simulink model "modelSVPWM"  (R2024a)
settings: Solver=ode23tb  StartTime=0.0  StopTime=0.1  MaxStep=sover_max_step  RelTol=1e-5
values from neighbouring files (symbols this model uses):
  f_fundamental = 265    [initBCPWM.m]    (also in initSVPWM.m = 100)
  f_pwm = 20000    [initBCPWM.m]    (also in initSVPWM.m)
  Ke = sqrt(2) * 3.35e-3 * 60 / 2 / pi / p    [initBCPWM.m]    (also in initSVPWM.m)
  load_angle = pi/6    (= 0.523598775598)    [initBCPWM.m]    (also in initSVPWM.m = load_angle_offset - voltage_angle)
  Ls = 3/2 * 1.2e-3    (= 0.0018)    [initBCPWM.m]    (also in initSVPWM.m)
  Rs = 3/2 * 0.8    (= 1.2)    [initBCPWM.m]    (also in initSVPWM.m)
  sover_max_step = 1e-6    (= 1e-06)    [initBCPWM.m]    (also in initSVPWM.m)
  V_uvw = Vsetpoint    (= 5)    [initSVPWM.m]
  Vdc = 24    [initBCPWM.m]    (also in initSVPWM.m)
libraries: simulink x14, spsSeriesRLCBranchLib x6, spsVoltageMeasurementLib x6, spsMosfetLib x6, spsNeutralLib x5, spsControlledVoltageSourceLib x3, spsCurrentMeasurementLib x3, spsGroundLib x2, spsDCVoltageSourceLib x1, spspowerguiLib x1
settings Model: Creator=mandr  LastModifiedBy=danielmcguiness
settings SolverCC: ZeroCrossControl=EnableAll  AlgebraicLoopSolver=TrustRegion  SolverResetMethod=Robust
settings DebuggingCC: UnconnectedInputMsg=warning  UnconnectedOutputMsg=warning  UnconnectedLineMsg=warning
settings ModelReferenceCC: EnableRefExpFcnMdlSchedulingChecks=on
settings RTWCC: GPUComputeCapability=3.5

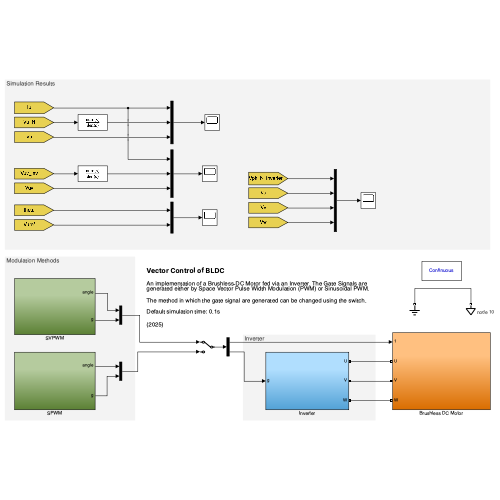
[thumbnail: Simulink's stored preview of the top-level diagram]
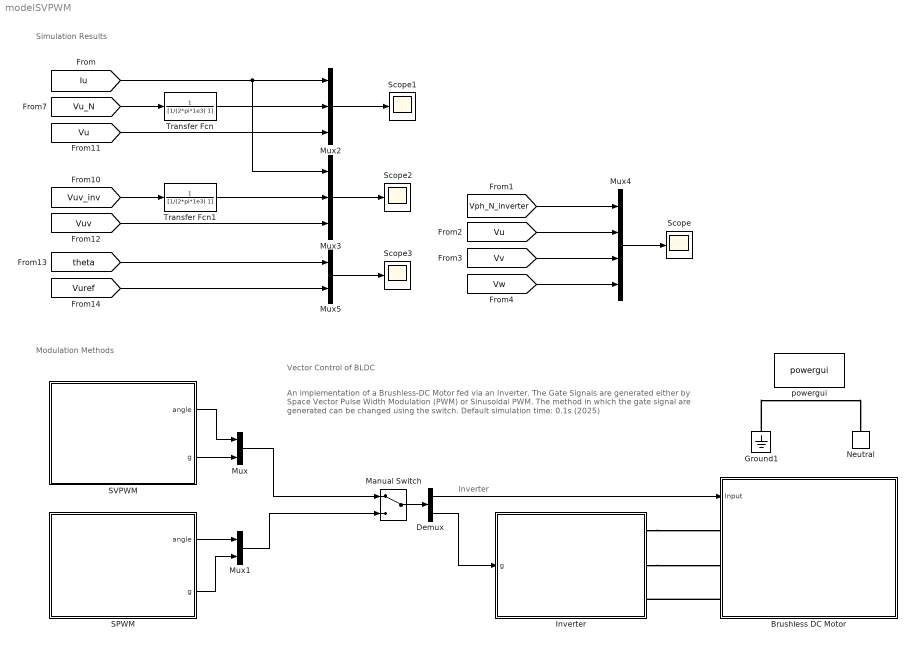
== system modelSVPWM ==
  note: Modulation Methods
  note: Simulation Results
  note: An implementation of a Brushless-DC Motor fed via an Inverter. The Gate Signals are generated either by Space Vector Pulse Width Modulation (PWM) or Sinusoidal PWM.
      |
      | The method in which the gate signal are generated can be changed using the switch.
      |
      | Default simulation time: 0.1s
      |
      | (2025)
  note: Vector Control of BLDC
  note: Inverter
  Brushless DC Motor : Subsystem
  Demux : Demux  Outputs=2
  Ground1 : spsGroundLib/Ground  LConnTagsString=a
  Inverter : Subsystem
  Manual Switch : ManualSwitch
  Mux : Mux  Inputs=2
  Mux1 : Mux  Inputs=2
  Mux2 : Mux  Inputs=3
  Mux3 : Mux  Inputs=3
  Mux4 : Mux
  Mux5 : Mux  Inputs=2
  Neutral : spsNeutralLib/Neutral  LConnTagsString=a  NodeNumber=10
      settings: AttributesFormatString=node %<NodeNumber>  LibrarySourceBlock=sps_lib/Utilities/Neutral
  SPWM : Subsystem
  SVPWM : Subsystem
  Scope{,1..3} (4 alike) : Scope
  Transfer Fcn : TransferFcn  Denominator=[1/(2*pi*1e3) 1]
  Transfer Fcn1 : TransferFcn  Denominator=[1/(2*pi*1e3) 1]
  powergui : spspowerguiLib/powergui  Priority=1  SimulationMode=Continuous  SampleTime=50e-6  frequency=60  Iterations=50  frequencyindice=0  Pbase=100e6  ErrMax=1e-4  UnitsV=kV  UnitsW=MW  buscounter=0  FunctionMessages=off  echomessages=off  EnableUseOfTLC=off  CurrentSourceSwitches=off  DisableSnubberDevices=off  DisableRonSwitches=off  DisableVfSwitches=off  DisplayEquations=off  AutomaticDiscreteSolvers=off  SolverType=Tustin/Backward Euler (TBE)  Interpol=off  ExternalGateDelay=off  methode=off  Ts=100  x0status=blocks  SPID=on  SwTol=0  HookPort=off  NonlinearTolerance=1e-4  nMaxIteration=100  ContinueOnMaxIteration=off  RestoreLinks=warning  ResistiveCurrentMeasurement=off  Frange=[0:2:500]  Ylog=off  Xlog=on  ShowGrid=off  save=off  variable=ZData  structure=0  ZoomFFT=off  StartTime=0.0  cycles=1  DisplayStyle=1  fundamental=60  FreqAxis=off  MaxFrequency=1000  frequencyindicesteady=1  RmsSteady=1  display=off
  wires:
  Mux/1 -> Manual Switch/1
  SVPWM/1(angle) -> Mux/1
  SVPWM/2(g) -> Mux/2
  Manual Switch/1 -> Demux/1
  Demux/2 -> Inverter/1(g)
  Demux/1 -> Brushless DC Motor/1(Input)
  SPWM/1(angle) -> Mux1/1
  SPWM/2(g) -> Mux1/2
  Mux1/1 -> Manual Switch/2
  [theta] -> Mux5/1
  Transfer Fcn/1 -> Mux2/2
  Mux2/1 -> Scope1/1
  [Vu_N] -> Transfer Fcn/1
  [Vuv] -> Mux3/3
  Transfer Fcn1/1 -> Mux3/2
  [Vuref] -> Mux5/2
  Mux3/1 -> Scope2/1
  [Vuv_inv] -> Transfer Fcn1/1
  [Vu] -> Mux2/3
  [Iu] -> Mux2/1, Mux3/1
  Mux4/1 -> Scope/1
  [Vw] -> Mux4/4
  [Vph_N_inverter] -> Mux4/1
  [Vv] -> Mux4/3
  [Vu] -> Mux4/2
  Mux5/1 -> Scope3/1
  connections:
  Inverter/RConn2 -- Brushless DC Motor/LConn2
  Brushless DC Motor/LConn3 -- Inverter/RConn3
  Inverter/RConn1 -- Brushless DC Motor/LConn1
  Ground1/LConn1 -- Neutral/LConn1

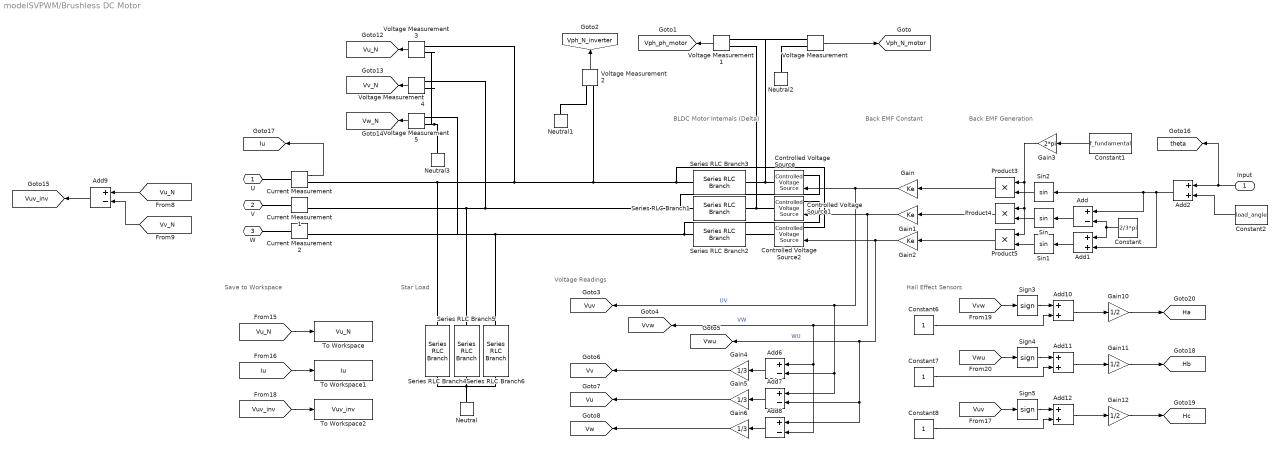
== system modelSVPWM/Brushless DC Motor ==
  note: Save to Workspace
  note: Star Load
  note: Back EMF Generation
  note: Back EMF Constant
  note: BLDC Motor Internals (Delta)
  note: Hall Effect Sensors
  note: Voltage Readings
  Input : Inport
  Add{,6..9} (5 alike) : Sum  Inputs=+-
  Add{1..2,10..12} (5 alike) : Sum
  Constant : Constant  Value=2/3*pi
  Constant1 : Constant  Value=f_fundamental
  Constant2 : Constant  Value=load_angle
  Constant6 : Constant
  Constant7 : Constant
  Constant8 : Constant
  Controlled Voltage Source : spsControlledVoltageSourceLib/Controlled Voltage Source  Initialize=on  Source_Type=AC  Amplitude=0  Phase=0  Frequency=0  Measurements=None
  Controlled Voltage Source1 : spsControlledVoltageSourceLib/Controlled Voltage Source  Initialize=on  Source_Type=AC  Amplitude=0  Phase=0  Frequency=0  Measurements=None
  Controlled Voltage Source2 : spsControlledVoltageSourceLib/Controlled Voltage Source  Initialize=on  Source_Type=AC  Amplitude=0  Phase=0  Frequency=0  Measurements=None
  Current Measurement : spsCurrentMeasurementLib/Current Measurement  PhasorSimulation=off  OutputType=Complex  PSBequivalent=0
  Current Measurement1 : spsCurrentMeasurementLib/Current Measurement  PhasorSimulation=off  OutputType=Complex  PSBequivalent=0
  Current Measurement2 : spsCurrentMeasurementLib/Current Measurement  PhasorSimulation=off  OutputType=Complex  PSBequivalent=0
  Gain : Gain  Gain=Ke
  Gain1 : Gain  Gain=Ke
  Gain10 : Gain  Gain=1/2
  Gain11 : Gain  Gain=1/2
  Gain12 : Gain  Gain=1/2
  Gain2 : Gain  Gain=Ke
  Gain3 : Gain  Gain=2*pi
  Gain4 : Gain  Gain=1/3
  Gain5 : Gain  Gain=1/3
  Gain6 : Gain  Gain=1/3
  Neutral{,1..3} (4 alike) : spsNeutralLib/Neutral  LConnTagsString=a  NodeNumber=10
      settings: AttributesFormatString=node %<NodeNumber>  LibrarySourceBlock=sps_lib/Utilities/Neutral
  Product3 : Product
  Product4 : Product
  Product5 : Product
  Series RLC Branch1 : spsSeriesRLCBranchLib/Series RLC Branch  LConnTagsString=__new0  RConnTagsString=__new0  BranchType=RL  Resistance=Rs  Inductance=Ls  SetiL0=off  InitialCurrent=0  Capacitance=1e-6  Setx0=off  InitialVoltage=0  Measurements=None
  Series RLC Branch2 : spsSeriesRLCBranchLib/Series RLC Branch  LConnTagsString=__new0  RConnTagsString=__new0  BranchType=RL  Resistance=Rs  Inductance=Ls  SetiL0=off  InitialCurrent=0  Capacitance=1e-6  Setx0=off  InitialVoltage=0  Measurements=None
  Series RLC Branch3 : spsSeriesRLCBranchLib/Series RLC Branch  LConnTagsString=__new0  RConnTagsString=__new0  BranchType=RL  Resistance=Rs  Inductance=Ls  SetiL0=off  InitialCurrent=0  Capacitance=1e-6  Setx0=off  InitialVoltage=0  Measurements=None
  Series RLC Branch4 : spsSeriesRLCBranchLib/Series RLC Branch  LConnTagsString=__new0  RConnTagsString=__new0  BranchType=R  Resistance=1e3  Inductance=Ls  SetiL0=off  InitialCurrent=0  Capacitance=1e-6  Setx0=off  InitialVoltage=0  Measurements=None
  Series RLC Branch5 : spsSeriesRLCBranchLib/Series RLC Branch  LConnTagsString=__new0  RConnTagsString=__new0  BranchType=R  Resistance=1e3  Inductance=Ls  SetiL0=off  InitialCurrent=0  Capacitance=1e-6  Setx0=off  InitialVoltage=0  Measurements=None
  Series RLC Branch6 : spsSeriesRLCBranchLib/Series RLC Branch  LConnTagsString=__new0  RConnTagsString=__new0  BranchType=R  Resistance=1e3  Inductance=Ls  SetiL0=off  InitialCurrent=0  Capacitance=1e-6  Setx0=off  InitialVoltage=0  Measurements=None
  Sign3 : Signum
  Sign4 : Signum
  Sign5 : Signum
  Sin : Trigonometry
  Sin1 : Trigonometry
  Sin2 : Trigonometry
  To Workspace : ToWorkspace  VariableName=Vu_N  SaveFormat=Timeseries  SampleTime=sover_max_step
  To Workspace1 : ToWorkspace  VariableName=Iu  SaveFormat=Timeseries  SampleTime=sover_max_step
  To Workspace2 : ToWorkspace  VariableName=Vuv_inv  SaveFormat=Timeseries  SampleTime=sover_max_step
  Voltage Measurement{,1..5} (6 alike) : spsVoltageMeasurementLib/Voltage Measurement  PhasorSimulation=off  OutputType=Complex  PSBequivalent=0
  U : PMIOPort  Side=Left
  V : PMIOPort  Port=2  Side=Left
  W : PMIOPort  Port=3  Side=Left
  tag scope: Ha=global, Hb=global, Hc=global, Iu=global, Vph_N_inverter=global, Vph_N_motor=global, Vph_ph_motor=global, Vu=global, Vu_N=global, Vuv=global, Vuv_inv=global, Vv=global, Vv_N=global, Vvw=global, Vw=global, Vw_N=global, Vwu=global, theta=global
  wires:
  Product5/1 -> Gain2/1
  Product3/1 -> Gain/1
  Constant/1 -> Add1/1, Add/2
  Product4/1 -> Gain1/1
  Add1/1 -> Sin1/1
  Add/1 -> Sin/1
  Sin2/1 -> Product3/2
  Sin/1 -> Product4/2
  Sin1/1 -> Product5/2
  Add2/1 -> Add1/2, Add/1, Sin2/1
  Constant1/1 -> Gain3/1
  Gain3/1 -> Product5/1, Product4/1, Product3/1
  Input/1 -> [theta], Add2/1
  Constant2/1 -> Add2/2
  Voltage Measurement/1 -> [Vph_N_motor]
  Voltage Measurement1/1 -> [Vph_ph_motor]
  Voltage Measurement2/1 -> [Vph_N_inverter]
  Current Measurement/1 -> [Iu]
  Voltage Measurement3/1 -> [Vu_N]
  Voltage Measurement4/1 -> [Vv_N]
  Voltage Measurement5/1 -> [Vw_N]
  [Vu_N] -> Add9/1
  [Vv_N] -> Add9/2
  Add9/1 -> [Vuv_inv]
  [Vu_N] -> To Workspace/1
  [Iu] -> To Workspace1/1
  [Vuv_inv] -> To Workspace2/1
  Add10/1 -> Gain10/1
  Sign4/1 -> Add11/1
  Constant6/1 -> Add10/2
  Gain10/1 -> [Ha]
  Sign3/1 -> Add10/1
  [Vvw] -> Sign3/1
  Sign5/1 -> Add12/1
  Add11/1 -> Gain11/1
  [Vwu] -> Sign4/1
  Gain12/1 -> [Hc]
  Constant7/1 -> Add11/2
  Gain11/1 -> [Hb]
  Add12/1 -> Gain12/1
  Constant8/1 -> Add12/2
  [Vuv] -> Sign5/1
  Add6/1 -> Gain4/1
  Add8/1 -> Gain6/1
  Add7/1 -> Gain5/1
  Gain1/1 -> Controlled Voltage Source1/1, Add8/2, Add6/1, [Vvw]  "VW"
  Gain4/1 -> [Vv]
  Gain2/1 -> Add8/1, Add7/2, [Vwu], Controlled Voltage Source2/1  "WU"
  Gain6/1 -> [Vw]
  Gain5/1 -> [Vu]
  Gain/1 -> [Vuv], Add7/1, Add6/2, Controlled Voltage Source/1  "UV"
  connections:
  Series RLC Branch4/LConn1 -- Current Measurement/RConn1 -- Voltage Measurement2/LConn1 -- Controlled Voltage Source2/LConn1 -- Series RLC Branch3/LConn1 -- Voltage Measurement3/LConn1
  Series RLC Branch5/LConn1 -- Current Measurement1/RConn1 -- Controlled Voltage Source/LConn1 -- Series RLC Branch1/LConn1 -- Voltage Measurement4/LConn1
  Series RLC Branch6/LConn1 -- Voltage Measurement5/LConn1 -- Current Measurement2/RConn1 -- Controlled Voltage Source1/LConn1 -- Series RLC Branch2/LConn1
  Series RLC Branch3/RConn1 -- Voltage Measurement/LConn1 -- Voltage Measurement1/LConn1 -- Controlled Voltage Source/RConn1
  Series RLC Branch1/RConn1 -- Voltage Measurement1/LConn2 -- Controlled Voltage Source1/RConn1
  Series RLC Branch2/RConn1 -- Controlled Voltage Source2/RConn1
  Series RLC Branch4/RConn1 -- Neutral/LConn1 -- Series RLC Branch5/RConn1 -- Series RLC Branch6/RConn1
  Voltage Measurement2/LConn2 -- Neutral1/LConn1
  Voltage Measurement/LConn2 -- Neutral2/LConn1
  U/RConn1 -- Current Measurement/LConn1
  Current Measurement1/LConn1 -- V/RConn1
  W/RConn1 -- Current Measurement2/LConn1
  Voltage Measurement5/LConn2 -- Voltage Measurement3/LConn2 -- Voltage Measurement4/LConn2 -- Neutral3/LConn1

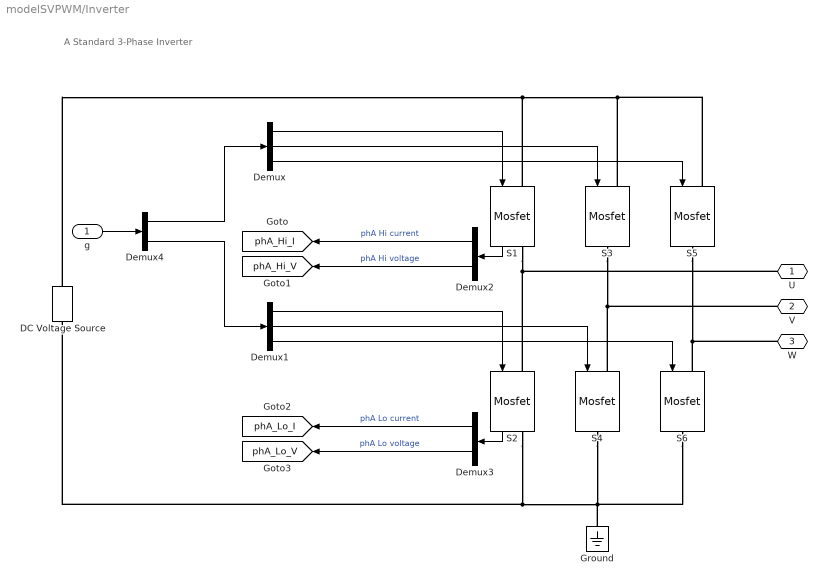
== system modelSVPWM/Inverter ==
  note: A Standard 3-Phase Inverter
  g : Inport
  DC Voltage Source : spsDCVoltageSourceLib/DC Voltage Source  Amplitude=Vdc  Measurements=None
  Demux : Demux  Outputs=3
  Demux1 : Demux  Outputs=3
  Demux2 : Demux  Outputs=2
  Demux3 : Demux  Outputs=2
  Demux4 : Demux  Outputs=2
  Ground : spsGroundLib/Ground  LConnTagsString=a
  S1 : spsMosfetLib/Mosfet  Ron=Ron  Lon=0  Rd=Rd  Vfd=Vf  IC=0  Rs=1e5  Cs=inf  Measurements=on
  S2 : spsMosfetLib/Mosfet  Ron=Ron  Lon=0  Rd=Rd  Vfd=Vf  IC=0  Rs=1e5  Cs=inf  Measurements=on
  S{3..6} (4 alike) : spsMosfetLib/Mosfet  Ron=Ron  Lon=0  Rd=Rd  Vfd=Vf  IC=0  Rs=1e5  Cs=inf  Measurements=off
  U : PMIOPort  Side=Right
  V : PMIOPort  Port=2  Side=Right
  W : PMIOPort  Port=3  Side=Right
  tag scope: phA_Hi_I=global, phA_Hi_V=global, phA_Lo_I=global, phA_Lo_V=global
  wires:
  Demux/3 -> S5/1
  Demux/1 -> S1/1
  Demux/2 -> S3/1
  Demux1/2 -> S4/1
  Demux1/1 -> S2/1
  Demux1/3 -> S6/1
  Demux3/1 -> [phA_Lo_I]  "phA Lo current"
  Demux3/2 -> [phA_Lo_V]  "phA Lo voltage"
  S2/1 -> Demux3/1
  S1/1 -> Demux2/1
  Demux2/1 -> [phA_Hi_I]  "phA Hi current"
  Demux2/2 -> [phA_Hi_V]  "phA Hi voltage"
  Demux4/1 -> Demux/1
  Demux4/2 -> Demux1/1
  g/1 -> Demux4/1
  connections:
  DC Voltage Source/RConn1 -- S5/LConn1 -- S3/LConn1 -- S1/LConn1
  S1/RConn1 -- S2/LConn1 -- U/RConn1
  DC Voltage Source/LConn1 -- S2/RConn1 -- S6/RConn1 -- Ground/LConn1 -- S4/RConn1
  W/RConn1 -- S6/LConn1 -- S5/RConn1
  V/RConn1 -- S3/RConn1 -- S4/LConn1

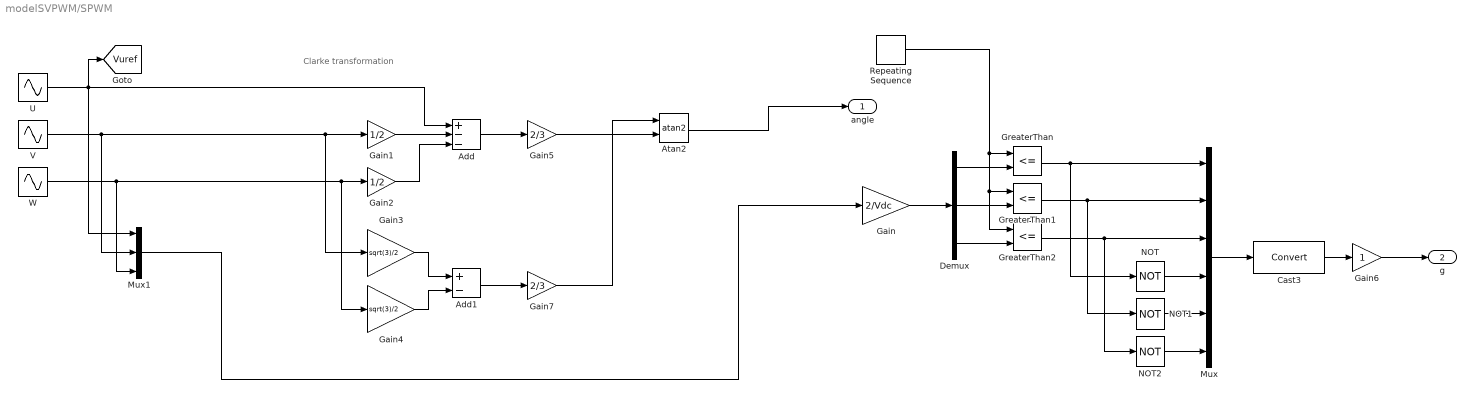
== system modelSVPWM/SPWM ==
  note: Clarke transformation
  Add : Sum  Inputs=+--
  Add1 : Sum  Inputs=+-
  Atan2 : Trigonometry  Operator=atan2
  Cast3 : DataTypeConversion  SaturateOnIntegerOverflow=off  RndMeth=Floor
  Demux : Demux  Outputs=3
  Gain : Gain  Gain=2/Vdc
  Gain1 : Gain  Gain=1/2
  Gain2 : Gain  Gain=1/2
  Gain3 : Gain  Gain=sqrt(3)/2
  Gain4 : Gain  Gain=sqrt(3)/2
  Gain5 : Gain  Gain=2/3
  Gain6 : Gain
  Gain7 : Gain  Gain=2/3
  GreaterThan : RelationalOperator  Operator=<=  OutDataTypeStr=boolean  RndMeth=Simplest  InputSameDT=off
  GreaterThan1 : RelationalOperator  Operator=<=  OutDataTypeStr=boolean  RndMeth=Simplest  InputSameDT=off
  GreaterThan2 : RelationalOperator  Operator=<=  OutDataTypeStr=boolean  RndMeth=Simplest  InputSameDT=off
  Mux : Mux  Inputs=6
  Mux1 : Mux  Inputs=3
  NOT : Logic  Operator=NOT  AllPortsSameDT=off  OutDataTypeStr=boolean
  NOT1 : Logic  Operator=NOT  AllPortsSameDT=off  OutDataTypeStr=boolean
  NOT2 : Logic  Operator=NOT  AllPortsSameDT=off  OutDataTypeStr=boolean
  Repeating Sequence : simulink/Sources/Repeating Sequence  rep_seq_t=[0 0.5/f_pwm 1/f_pwm]  rep_seq_y=[-1 1 -1]
  U : Sin  Amplitude=V_uvw  Frequency=2*pi*f_fundamental  SampleTime=0
  V : Sin  Amplitude=V_uvw  Frequency=2*pi*f_fundamental  Phase=-2*pi/3  SampleTime=0
  W : Sin  Amplitude=V_uvw  Frequency=2*pi*f_fundamental  Phase=2*pi/3  SampleTime=0
  angle : Outport
  g : Outport  Port=2
  tag scope: Vuref=global
  wires:
  Mux/1 -> Cast3/1
  NOT/1 -> Mux/4
  NOT2/1 -> Mux/6
  NOT1/1 -> Mux/5
  Cast3/1 -> Gain6/1
  Gain6/1 -> g/1
  Atan2/1 -> angle/1
  Mux1/1 -> Gain/1
  Gain/1 -> Demux/1
  Repeating Sequence/1 -> GreaterThan2/1, GreaterThan1/1, GreaterThan/1
  Demux/1 -> GreaterThan/2
  Demux/2 -> GreaterThan1/2
  Demux/3 -> GreaterThan2/2
  GreaterThan/1 -> NOT/1, Mux/1
  GreaterThan1/1 -> Mux/2, NOT1/1
  GreaterThan2/1 -> NOT2/1, Mux/3
  Gain7/1 -> Atan2/1
  Add/1 -> Gain5/1
  V/1 -> Mux1/2, Gain3/1, Gain1/1
  Gain1/1 -> Add/2
  W/1 -> Mux1/3, Gain4/1, Gain2/1
  Gain4/1 -> Add1/2
  Gain2/1 -> Add/3
  Gain5/1 -> Atan2/2
  U/1 -> [Vuref], Mux1/1, Add/1
  Gain3/1 -> Add1/1
  Add1/1 -> Gain7/1

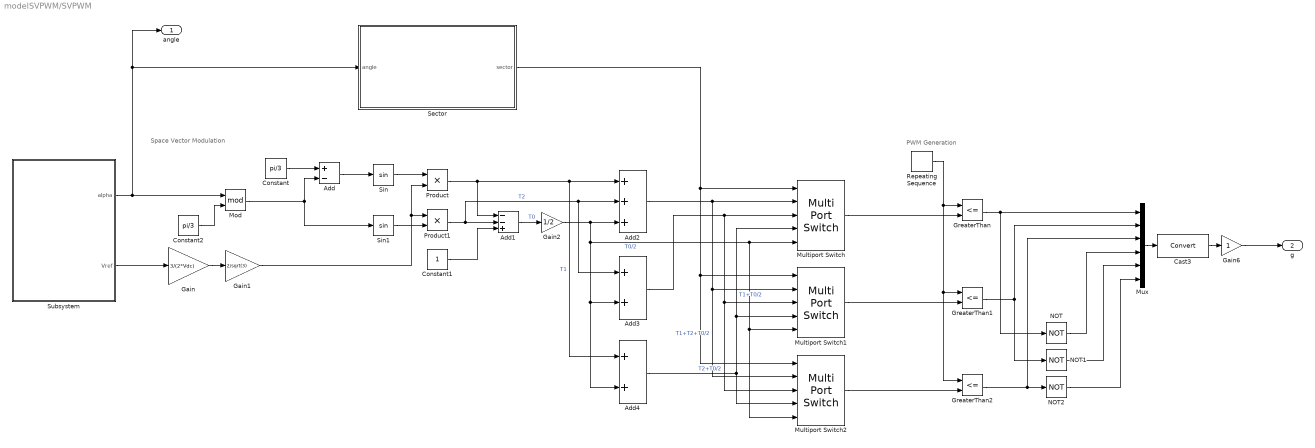
== system modelSVPWM/SVPWM ==
  note: PWM Generation
  note: Space Vector Modulation
  Add : Sum  Inputs=+-
  Add1 : Sum  Inputs=--+
  Add2 : Sum  Inputs=+++
  Add3 : Sum
  Add4 : Sum
  Cast3 : DataTypeConversion  SaturateOnIntegerOverflow=off  RndMeth=Floor
  Constant : Constant  Value=pi/3
  Constant1 : Constant
  Constant2 : Constant  Value=pi/3
  Gain : Gain  Gain=3/(2*Vdc)
  Gain1 : Gain  Gain=2/sqrt(3)
  Gain2 : Gain  Gain=1/2
  Gain6 : Gain
  GreaterThan : RelationalOperator  Operator=<=  OutDataTypeStr=boolean  RndMeth=Simplest  InputSameDT=off
  GreaterThan1 : RelationalOperator  Operator=<=  OutDataTypeStr=boolean  RndMeth=Simplest  InputSameDT=off
  GreaterThan2 : RelationalOperator  Operator=<=  OutDataTypeStr=boolean  RndMeth=Simplest  InputSameDT=off
  Mod : Math  Operator=mod
  Multiport Switch : MultiPortSwitch  DataPortOrder=Specify indices  DataPortIndices={[1,6],5,2,[3,4]}  SaturateOnIntegerOverflow=off  InputSameDT=off
  Multiport Switch1 : MultiPortSwitch  DataPortOrder=Specify indices  DataPortIndices={[2,3],1,4,[5,6]}  SaturateOnIntegerOverflow=off  InputSameDT=off
  Multiport Switch2 : MultiPortSwitch  DataPortOrder=Specify indices  DataPortIndices={[4,5],3,6,[1,2]}  SaturateOnIntegerOverflow=off  InputSameDT=off
  Mux : Mux  Inputs=6
  NOT : Logic  Operator=NOT  AllPortsSameDT=off  OutDataTypeStr=boolean
  NOT1 : Logic  Operator=NOT  AllPortsSameDT=off  OutDataTypeStr=boolean
  NOT2 : Logic  Operator=NOT  AllPortsSameDT=off  OutDataTypeStr=boolean
  Product : Product
  Product1 : Product
  Repeating Sequence : simulink/Sources/Repeating Sequence  rep_seq_t=[0 0.5/f_pwm 1/f_pwm]  rep_seq_y=[0 1 0]
  Sector : Subsystem
  Sin : Trigonometry
  Sin1 : Trigonometry
  Subsystem : Subsystem
  angle : Outport
  g : Outport  Port=2
  wires:
  Sin1/1 -> Product1/2
  Gain1/1 -> Product1/1, Product/2
  Repeating Sequence/1 -> GreaterThan2/1, GreaterThan1/1, GreaterThan/1
  Add1/1 -> Gain2/1  "T0"
  Sector/1(sector) -> Multiport Switch/1, Multiport Switch2/1, Multiport Switch1/1
  Gain2/1 -> Add2/3, Multiport Switch2/5, Multiport Switch1/5, Multiport Switch/5, Add3/2, Add4/2  "T0/2"
  Mod/1 -> Add/2, Sin1/1
  Add4/1 -> Multiport Switch/4, Multiport Switch1/4, Multiport Switch2/4  "T1+T0/2"
  Add3/1 -> Multiport Switch2/3, Multiport Switch1/3, Multiport Switch/3  "T2+T0/2"
  Multiport Switch1/1 -> GreaterThan1/2
  Add2/1 -> Multiport Switch2/2, Multiport Switch1/2, Multiport Switch/2  "T1+T2+T0/2"
  Mux/1 -> Cast3/1
  Constant/1 -> Add/1
  Product/1 -> Add2/1, Add4/1, Add1/1  "T1"
  Subsystem/1(alpha) -> Mod/1, angle/1, Sector/1(angle)
  NOT/1 -> Mux/4
  Product1/1 -> Add1/2, Add2/2, Add3/1  "T2"
  Sin/1 -> Product/1
  Add/1 -> Sin/1
  NOT2/1 -> Mux/6
  Gain/1 -> Gain1/1
  Constant2/1 -> Mod/2
  Constant1/1 -> Add1/3
  Subsystem/2(Vref) -> Gain/1
  Multiport Switch/1 -> GreaterThan/2
  Multiport Switch2/1 -> GreaterThan2/2
  NOT1/1 -> Mux/5
  Cast3/1 -> Gain6/1
  Gain6/1 -> g/1
  GreaterThan/1 -> NOT/1, Mux/1
  GreaterThan1/1 -> NOT1/1, Mux/2
  GreaterThan2/1 -> NOT2/1, Mux/3

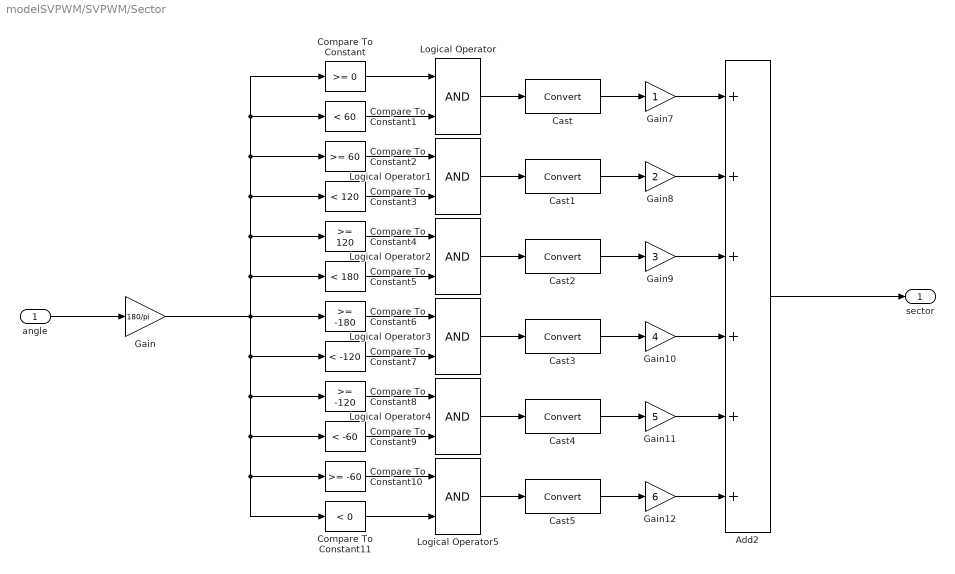
== system modelSVPWM/SVPWM/Sector ==
  angle : Inport
  Add2 : Sum  Inputs=6
  Cast{,1..5} (6 alike) : DataTypeConversion  SaturateOnIntegerOverflow=off  RndMeth=Floor
  Compare To Constant : simulink/Logic and Bit Operations/Compare To Constant  relop=>=  const=0  OutDataTypeStr=boolean
  Compare To Constant1 : simulink/Logic and Bit Operations/Compare To Constant  relop=<  const=60  OutDataTypeStr=boolean
  Compare To Constant10 : simulink/Logic and Bit Operations/Compare To Constant  relop=>=  const=-60  OutDataTypeStr=boolean
  Compare To Constant11 : simulink/Logic and Bit Operations/Compare To Constant  relop=<  const=0  OutDataTypeStr=boolean
  Compare To Constant2 : simulink/Logic and Bit Operations/Compare To Constant  relop=>=  const=60  OutDataTypeStr=boolean
  Compare To Constant3 : simulink/Logic and Bit Operations/Compare To Constant  relop=<  const=120  OutDataTypeStr=boolean
  Compare To Constant4 : simulink/Logic and Bit Operations/Compare To Constant  relop=>=  const=120  OutDataTypeStr=boolean
  Compare To Constant5 : simulink/Logic and Bit Operations/Compare To Constant  relop=<  const=180  OutDataTypeStr=boolean
  Compare To Constant6 : simulink/Logic and Bit Operations/Compare To Constant  relop=>=  const=-180  OutDataTypeStr=boolean
  Compare To Constant7 : simulink/Logic and Bit Operations/Compare To Constant  relop=<  const=-120  OutDataTypeStr=boolean
  Compare To Constant8 : simulink/Logic and Bit Operations/Compare To Constant  relop=>=  const=-120  OutDataTypeStr=boolean
  Compare To Constant9 : simulink/Logic and Bit Operations/Compare To Constant  relop=<  const=-60  OutDataTypeStr=boolean
  Gain : Gain  Gain=180/pi
  Gain10 : Gain  Gain=4
  Gain11 : Gain  Gain=5
  Gain12 : Gain  Gain=6
  Gain7 : Gain
  Gain8 : Gain  Gain=2
  Gain9 : Gain  Gain=3
  Logical Operator{,1..5} (6 alike) : Logic  AllPortsSameDT=off  OutDataTypeStr=boolean
  sector : Outport
  wires:
  Cast3/1 -> Gain10/1
  Gain9/1 -> Add2/3
  Logical Operator2/1 -> Cast2/1
  Logical Operator3/1 -> Cast3/1
  Compare To Constant11/1 -> Logical Operator5/2
  Compare To Constant2/1 -> Logical Operator1/1
  Cast2/1 -> Gain9/1
  angle/1 -> Gain/1
  Gain7/1 -> Add2/1
  Gain10/1 -> Add2/4
  Gain12/1 -> Add2/6
  Compare To Constant3/1 -> Logical Operator1/2
  Compare To Constant7/1 -> Logical Operator3/2
  Compare To Constant6/1 -> Logical Operator3/1
  Cast/1 -> Gain7/1
  Cast5/1 -> Gain12/1
  Compare To Constant8/1 -> Logical Operator4/1
  Cast4/1 -> Gain11/1
  Cast1/1 -> Gain8/1
  Gain8/1 -> Add2/2
  Add2/1 -> sector/1
  Compare To Constant4/1 -> Logical Operator2/1
  Compare To Constant/1 -> Logical Operator/1
  Logical Operator/1 -> Cast/1
  Compare To Constant1/1 -> Logical Operator/2
  Compare To Constant5/1 -> Logical Operator2/2
  Compare To Constant9/1 -> Logical Operator4/2
  Logical Operator4/1 -> Cast4/1
  Logical Operator5/1 -> Cast5/1
  Compare To Constant10/1 -> Logical Operator5/1
  Logical Operator1/1 -> Cast1/1
  Gain11/1 -> Add2/5
  Gain/1 -> Compare To Constant8/1, Compare To Constant10/1, Compare To Constant11/1, Compare To Constant9/1, Compare To Constant7/1, Compare To Constant/1, Compare To Constant1/1, Compare To Constant2/1, Compare To Constant3/1, Compare To Constant4/1, Compare To Constant5/1, Compare To Constant6/1

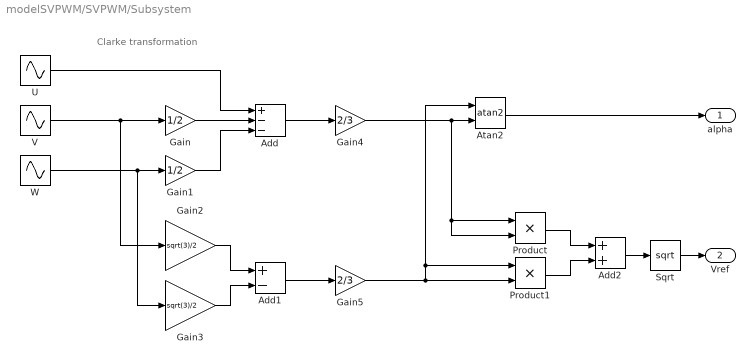
== system modelSVPWM/SVPWM/Subsystem ==
  note: Clarke transformation
  Add : Sum  Inputs=+--
  Add1 : Sum  Inputs=+-
  Add2 : Sum
  Atan2 : Trigonometry  Operator=atan2
  Gain : Gain  Gain=1/2
  Gain1 : Gain  Gain=1/2
  Gain2 : Gain  Gain=sqrt(3)/2
  Gain3 : Gain  Gain=sqrt(3)/2
  Gain4 : Gain  Gain=2/3
  Gain5 : Gain  Gain=2/3
  Product : Product
  Product1 : Product
  Sqrt : Sqrt
  U : Sin  Amplitude=V_uvw  Frequency=2*pi*f_fundamental  SampleTime=0
  V : Sin  Amplitude=V_uvw  Frequency=2*pi*f_fundamental  Phase=-2*pi/3  SampleTime=0
  W : Sin  Amplitude=V_uvw  Frequency=2*pi*f_fundamental  Phase=2*pi/3  SampleTime=0
  alpha : Outport
  Vref : Outport  Port=2
  wires:
  W/1 -> Gain3/1, Gain1/1
  Gain/1 -> Add/2
  Gain2/1 -> Add1/1
  Gain5/1 -> Atan2/1, Product1/1, Product1/2
  Gain1/1 -> Add/3
  U/1 -> Add/1
  Add/1 -> Gain4/1
  Add1/1 -> Gain5/1
  V/1 -> Gain2/1, Gain/1
  Gain3/1 -> Add1/2
  Gain4/1 -> Product/2, Product/1, Atan2/2
  Atan2/1 -> alpha/1
  Product/1 -> Add2/1
  Product1/1 -> Add2/2
  Add2/1 -> Sqrt/1
  Sqrt/1 -> Vref/1
